simulink model "model_template_for_report_R2015b"  (R2016a)
settings: Solver=VariableStepAuto  SolverMode=SingleTasking  StartTime=0.0  StopTime=5  RelTol=1e-3
values from neighbouring files (symbols this model uses):
  den = [1/(avgwn^2) 2*avgeps/avgwn 1]    [main.m]
  k = 0.21763    [main.m]    (also in rootlocus.m = 92)
  num = avgq    [main.m]
  poles = [0]    [main.m]
  zeroes = [-35.99]    [main.m]
undefined symbols (not defined in the file or in its folder): zp, zz
libraries: simulink x1
settings Model: Creator=simon  LastModifiedBy=mehetab
settings SolverCC: ZeroCrossControl=DisableAll
settings DebuggingCC: SFUnexpectedBacktrackingDiag=error  SFNoUnconditionalDefaultTransitionDiag=error
settings GRTTargetCC: TargetLangStandard=C99 (ISO)  GeneratePreprocessorConditionals=Use local settings
settings ConfigComp: CovMetricSettings=dwe  CovHtmlReporting=off  CovSaveCumulativeToWorkspaceVar=off  CovSaveSingleToWorkspaceVar=off  CovModelRefEnable=Off  CovExternalEMLEnable=on

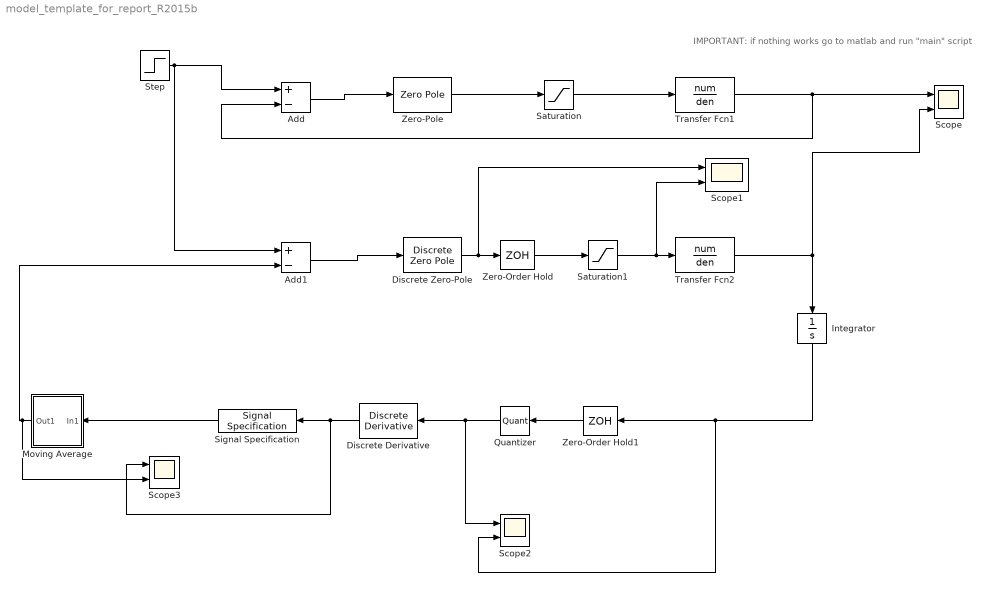
== system model_template_for_report_R2015b ==
  note: IMPORTANT: if nothing works go to matlab and run "main" script
  Add : Sum  Inputs=+-
  Add1 : Sum  Inputs=+-
  Discrete Zero-Pole : DiscreteZeroPole  Zeros=zz  Poles=zp  Gain=k  SampleTime=0.002
  Discrete Derivative : simulink/Discrete/Discrete Derivative  gainval=1.0  ICPrevScaledInput=0.0  OutMin=[]  OutMax=[]  OutDataType=fixdt(1, 16)  OutScaling=2^-10  DoSatur=off
  Integrator : Integrator
  Moving Average : Subsystem  Description=Replaced Block  mask(Replaced Block){}
      mask help: This block has been replaced with an empty subsystem because it used functionality that is unavailable in Simulink R2015b.
      mask Display: fprintf('Replaced: %s\n','dspstat3/Moving Average')
  Quantizer : Quantizer  QuantizationInterval=0.01*pi/180
  Saturation : Saturate  UpperLimit=1  LowerLimit=-1
  Saturation1 : Saturate  UpperLimit=1  LowerLimit=-1  LinearizeAsGain=off
  Scope{,1..3} (4 alike) : Scope  NumInputPorts=2
  Signal Specification : SignalSpecification  Dimensions=1  SampleTime=0.002
  Step : Step  After=0.5  SampleTime=0
  Transfer Fcn1 : TransferFcn  Numerator=num  Denominator=den
  Transfer Fcn2 : TransferFcn  Numerator=num  Denominator=den
  Zero-Order Hold : ZeroOrderHold  SampleTime=0.002
  Zero-Order Hold1 : ZeroOrderHold  SampleTime=0.002
  Zero-Pole : ZeroPole  Zeros=zeroes  Poles=poles  Gain=k
  wires:
  Add/1 -> Zero-Pole/1
  Zero-Pole/1 -> Saturation/1
  Saturation/1 -> Transfer Fcn1/1
  Add1/1 -> Discrete Zero-Pole/1
  Step/1 -> Add1/1, Add/1
  Saturation1/1 -> Scope1/2, Transfer Fcn2/1
  Discrete Zero-Pole/1 -> Scope1/1, Zero-Order Hold/1
  Transfer Fcn2/1 -> Integrator/1, Scope/2
  Zero-Order Hold/1 -> Saturation1/1
  Transfer Fcn1/1 -> Add/2, Scope/1
  Integrator/1 -> Scope2/2, Zero-Order Hold1/1
  Zero-Order Hold1/1 -> Quantizer/1
  Quantizer/1 -> Scope2/1, Discrete Derivative/1
  Discrete Derivative/1 -> Scope3/1, Signal Specification/1
  Signal Specification/1 -> Moving Average/1(In1)
  Moving Average/1(Out1) -> Scope3/2, Add1/2

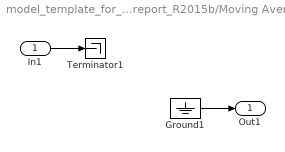
== system model_template_for_report_R2015b/Moving Average ==
  In1 : Inport
  Ground1 : Ground
  Terminator1 : Terminator
  Out1 : Outport
  wires:
  Ground1/1 -> Out1/1
  In1/1 -> Terminator1/1
